simulink model "solved_navigation_function_R2017a"  (R2017a)
settings: Solver=ode45  StartTime=0.0  StopTime=simulation_time  MaxStep=0.01  RelTol=1e-3  EnableMultiTasking=on
undefined symbols (not defined in the file): parameters, path_to_track, sampling_time, x0
settings Model: Creator=ezequiel  LastModifiedBy=ezequiel
settings OptimizationCC: LifeSpan=inf
settings DebuggingCC: AllowSymbolicDim=off  SFUnexpectedBacktrackingDiag=warning  SFNoUnconditionalDefaultTransitionDiag=warning  SFExecutionAtInitializationDiag=none
settings ModelReferenceCC: PropagateSignalLabelsOutOfModel=off
settings GRTTargetCC: TargetLangStandard=C89/C90 (ANSI)
settings ConfigComp: CovMetricSettings=dw  CovHtmlReporting=on  CovSaveCumulativeToWorkspaceVar=on  CovSaveSingleToWorkspaceVar=on  CovExternalEMLEnable=off

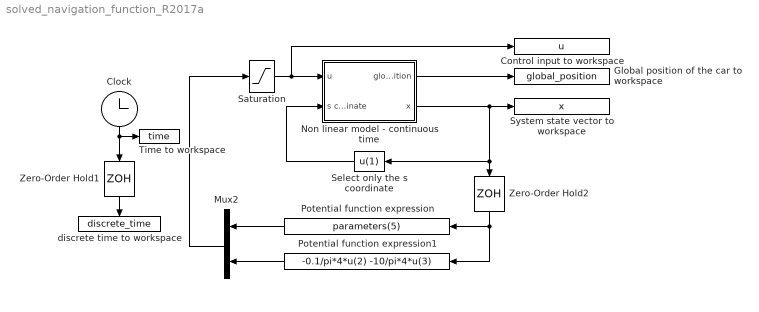
== system solved_navigation_function_R2017a ==
  Clock : Clock
  Control input to workspace : ToWorkspace  VariableName=u  SampleTime=-1
  Global position of the car to workspace : ToWorkspace  VariableName=global_position  SampleTime=-1
  Mux2 : Mux  Inputs=2
  Non linear model - continuous time : Subsystem
  Potential function expression : Fcn  Expr=parameters(5)
  Potential function expression1 : Fcn  Expr=-0.1/pi*4*u(2) -10/pi*4*u(3)
  Saturation : Saturate  UpperLimit=[Inf;pi/4]  LowerLimit=[0;-pi/4]
  Select only the s coordinate : Fcn  Expr=u(1)
  System state vector to workspace : ToWorkspace  VariableName=x  SampleTime=-1
  Time to workspace : ToWorkspace  VariableName=time  SampleTime=-1
  Zero-Order Hold1 : ZeroOrderHold  SampleTime=sampling_time
  Zero-Order Hold2 : ZeroOrderHold  SampleTime=sampling_time
  discrete time to workspace : ToWorkspace  VariableName=discrete_time  SampleTime=-1
  wires:
  Non linear model - continuous time/2(x) -> System state vector to workspace/1, Select only the s coordinate/1, Zero-Order Hold2/1
  Non linear model - continuous time/1(global_position) -> Global position of the car to workspace/1
  Select only the s coordinate/1 -> Non linear model - continuous time/2(s coordinate)
  Saturation/1 -> Non linear model - continuous time/1(u), Control input to workspace/1
  Mux2/1 -> Saturation/1
  Zero-Order Hold2/1 -> Potential function expression/1, Potential function expression1/1
  Potential function expression/1 -> Mux2/1
  Potential function expression1/1 -> Mux2/2
  Clock/1 -> Zero-Order Hold1/1, Time to workspace/1
  Zero-Order Hold1/1 -> discrete time to workspace/1

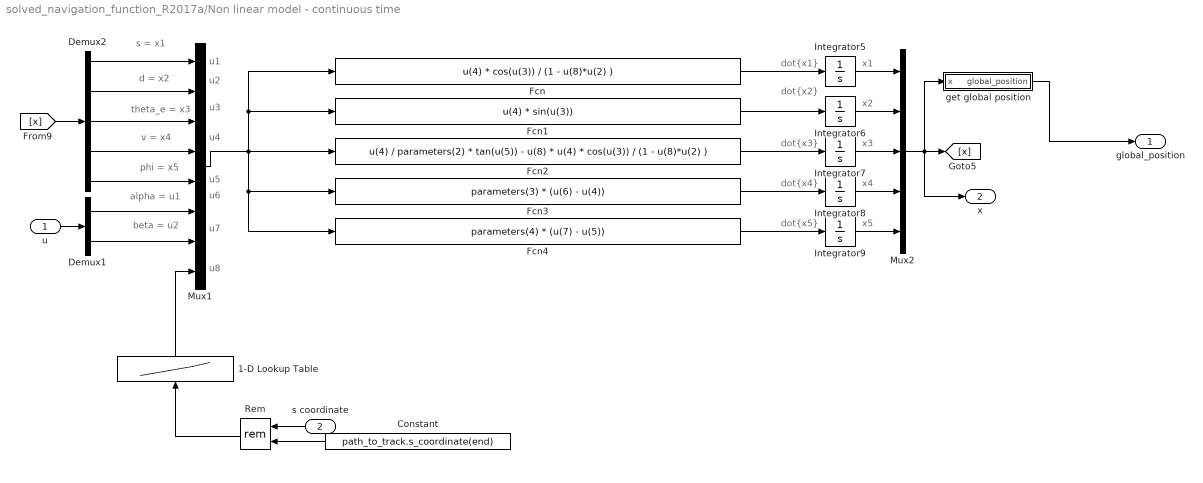
== system solved_navigation_function_R2017a/Non linear model - continuous time ==
  note: s = x1
  note: dot{x1}
  note: d = x2
  note: theta_e = x3
  note: v = x4
  note: phi = x5
  note: alpha = u1
  note: beta = u2
  note: u1
  note: u2
  note: u3
  note: u4
  note: u5
  note: u6
  note: u7
  note: x1
  note: dot{x2}
  note: x2
  note: dot{x3}
  note: x3
  note: dot{x4}
  note: x4
  note: dot{x5}
  note: x5
  note: u8
  u : Inport
  s coordinate : Inport  Port=2
  1-D Lookup Table : Lookup_n-D  NumberOfTableDimensions=1  BreakpointsForDimension1=path_to_track.s_coordinate  Table=path_to_track.curvature  InternalRulePriority=Speed  RndMeth=Simplest  InputSameDT=on
  Constant : Constant  Value=path_to_track.s_coordinate(end)
  Demux1 : Demux  Outputs=2
  Demux2 : Demux  Outputs=5
  Fcn : Fcn  Expr=u(4) * cos(u(3)) / (1 - u(8)*u(2) )
  Fcn1 : Fcn  Expr=u(4) * sin(u(3))
  Fcn2 : Fcn  Expr=u(4) / parameters(2) * tan(u(5)) - u(8) * u(4) * cos(u(3)) / (1 - u(8)*u(2) )
  Fcn3 : Fcn  Expr=parameters(3) * (u(6) - u(4))
  Fcn4 : Fcn  Expr=parameters(4) * (u(7) - u(5))
  Integrator5 : Integrator  InitialCondition=x0(1)
  Integrator6 : Integrator  InitialCondition=x0(2)
  Integrator7 : Integrator  InitialCondition=x0(3)
  Integrator8 : Integrator  InitialCondition=x0(4)
  Integrator9 : Integrator  InitialCondition=x0(5)
  Mux1 : Mux  Inputs=8
  Mux2 : Mux  Inputs=5
  Rem : Math  Operator=rem  SaturateOnIntegerOverflow=on
  get global position : Subsystem
  global_position : Outport
  x : Outport  Port=2
  wires:
  u/1 -> Demux1/1
  Fcn/1 -> Integrator5/1
  Demux2/1 -> Mux1/1
  Demux2/2 -> Mux1/2
  Demux2/3 -> Mux1/3
  Demux2/4 -> Mux1/4
  Demux2/5 -> Mux1/5
  Demux1/1 -> Mux1/6
  Demux1/2 -> Mux1/7
  Mux1/1 -> Fcn3/1, Fcn4/1, Fcn1/1, Fcn/1, Fcn2/1
  Fcn1/1 -> Integrator6/1
  Integrator6/1 -> Mux2/2
  Fcn2/1 -> Integrator7/1
  Integrator7/1 -> Mux2/3
  Fcn3/1 -> Integrator8/1
  Integrator8/1 -> Mux2/4
  Fcn4/1 -> Integrator9/1
  Integrator9/1 -> Mux2/5
  [x] -> Demux2/1
  Integrator5/1 -> Mux2/1
  1-D Lookup Table/1 -> Mux1/8
  Rem/1 -> 1-D Lookup Table/1
  Constant/1 -> Rem/2
  s coordinate/1 -> Rem/1
  Mux2/1 -> get global position/1(x), x/1, [x]
  get global position/1(global_position) -> global_position/1

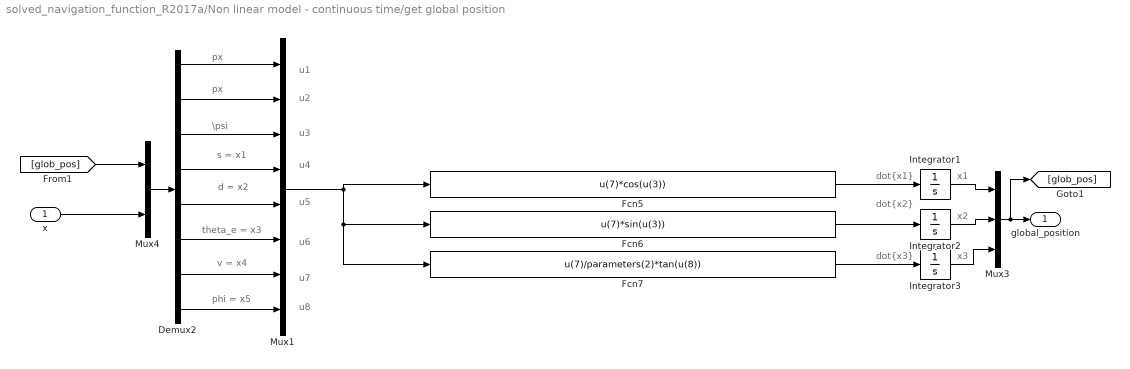
== system solved_navigation_function_R2017a/Non linear model - continuous time/get global position ==
  note: s = x1
  note: d = x2
  note: theta_e = x3
  note: v = x4
  note: phi = x5
  note: u1
  note: u2
  note: u3
  note: u4
  note: u5
  note: u6
  note: u7
  note: px
  note: px
  note: \psi
  note: u8
  note: x2
  note: x1
  note: dot{x2}
  note: dot{x1}
  note: dot{x3}
  note: x3
  x : Inport
  Demux2 : Demux  Outputs=8
  Fcn5 : Fcn  Expr=u(7)*cos(u(3))
  Fcn6 : Fcn  Expr=u(7)*sin(u(3))
  Fcn7 : Fcn  Expr=u(7)/parameters(2)*tan(u(8))
  Integrator1 : Integrator
  Integrator2 : Integrator
  Integrator3 : Integrator
  Mux1 : Mux  Inputs=8
  Mux3 : Mux  Inputs=3
  Mux4 : Mux  Inputs=2
  global_position : Outport
  wires:
  Mux1/1 -> Fcn7/1, Fcn6/1, Fcn5/1
  x/1 -> Mux4/2
  Demux2/1 -> Mux1/1
  Demux2/2 -> Mux1/2
  Demux2/3 -> Mux1/3
  Demux2/4 -> Mux1/4
  Demux2/5 -> Mux1/5
  Demux2/6 -> Mux1/6
  Demux2/7 -> Mux1/7
  Demux2/8 -> Mux1/8
  Fcn6/1 -> Integrator2/1
  Integrator2/1 -> Mux3/2
  Fcn5/1 -> Integrator1/1
  Integrator3/1 -> Mux3/3
  Integrator1/1 -> Mux3/1
  Fcn7/1 -> Integrator3/1
  Mux3/1 -> [glob_pos], global_position/1
  [glob_pos] -> Mux4/1
  Mux4/1 -> Demux2/1
